simulink model "D2C_boucle_vitesse_modelisation"  (R2018a)
settings: Solver=ode45  StartTime=0.0  StopTime=6  FixedStep=0.003  RelTol=1e-3  EnableMultiTasking=on
settings Model: Creator=Propriétaire  LastModifiedBy=emiliendurif
settings DataIOCC: LimitDataPoints=on  SaveFormat=Array  SignalLoggingSaveFormat=ModelDataLogs
settings OptimizationCC: ExpressionDepthLimit=2147483647  LifeSpan=inf
settings DebuggingCC: UnderspecifiedInitializationDetection=Classic  MergeDetectMultiDrivingBlocksExec=none  SolverPrmCheckMsg=warning  FcnCallInpInsideContextMsg=warning  StateNameClashWarn=warning  SFUnexpectedBacktrackingDiag=warning  SFNoUnconditionalDefaultTransitionDiag=warning  SFExecutionAtInitializationDiag=none
settings HardwareCC: ProdBitPerPointer=32  ProdBitPerSizeT=32  ProdBitPerPtrDiffT=32  ProdLargestAtomicFloat=None  ProdIntDivRoundTo=Undefined  ProdEndianess=Unspecified  ProdWordSize=32  ProdHWDeviceType=32-bit Generic
settings ModelReferenceCC: PropagateSignalLabelsOutOfModel=off
settings CodeAppCC: StateflowObjectComments=on
settings GRTTargetCC: TargetLangStandard=C89/C90 (ANSI)  GeneratePreprocessorConditionals=Disable all  CombineOutputUpdateFcns=off  GRTInterface=on
settings ConfigComp: CovMetricSettings=dw  CovHtmlReporting=on  CovSaveCumulativeToWorkspaceVar=on  CovSaveSingleToWorkspaceVar=on  CovExternalEMLEnable=off

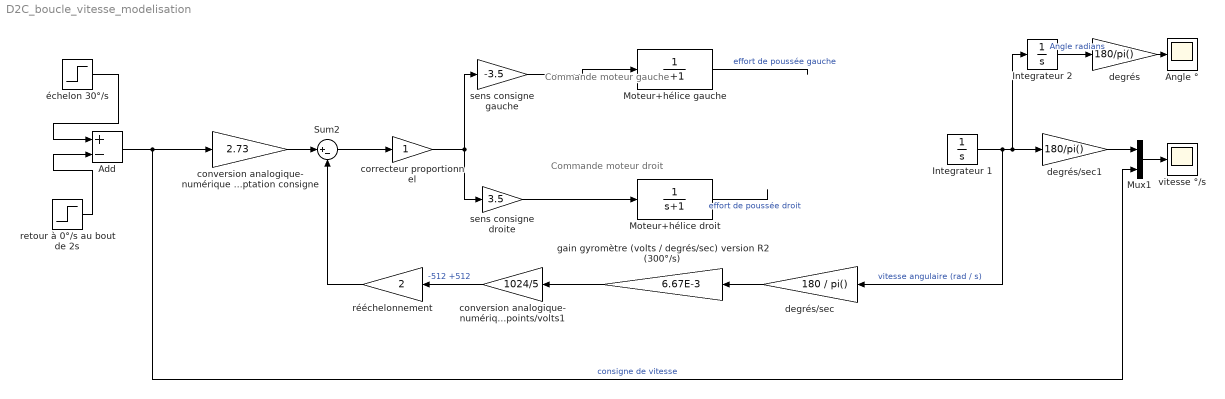
== system D2C_boucle_vitesse_modelisation ==
  note: Commande
      | moteur gauche
  note: Commande
      | moteur droit
  Add : Sum  Inputs=+-
  Angle ° : Scope
  Integrateur 1 : Integrator
  Integrateur 2 : Integrator
  Moteur+hélice droit : TransferFcn  Denominator=[1 1]
  Moteur+hélice gauche : TransferFcn  Denominator=[1 1]
  Mux1 : Mux  Inputs=2
  Sum2 : Sum  Inputs=|+-
  conversion analogique- numérique points/volts 15 bits et adaptation consigne : Gain  Gain=2.73
  conversion analogique- numérique points/volts1 : Gain  Gain=1024/5
  correcteur proportionnel : Gain
  degrés : Gain  Gain=180/pi()
  degrés/sec : Gain  Gain=180 / pi()
  degrés/sec1 : Gain  Gain=180/pi()
  gain gyromètre (volts / degrés/sec) version R2 (300°/s) : Gain  Gain=6.67E-3
  retour à 0°/s au bout de 2s : Step  Time=2  After=30  SampleTime=0
  rééchelonnement : Gain  Gain=2
  sens consigne droite : Gain  Gain=3.5
  sens consigne gauche : Gain  Gain=-3.5
  vitesse °/s : Scope
  échelon 30°/s : Step  Time=0  After=30  SampleTime=0
  wires:
  Moteur+hélice gauche/1 -> ?  "effort de poussée gauche"
  Moteur+hélice droit/1 -> ?  "effort de poussée droit"
  gain gyromètre (volts / degrés/sec) version R2 (300°/s)/1 -> conversion analogique- numérique points/volts1/1
  Integrateur 2/1 -> degrés/1  "Angle radians"
  ? -> Integrateur 1/1  "accélération angulaire"
  Integrateur 1/1 -> Integrateur 2/1, degrés/sec1/1, degrés/sec/1  "vitesse angulaire (rad / s)"
  degrés/sec/1 -> gain gyromètre (volts / degrés/sec) version R2 (300°/s)/1
  degrés/1 -> Angle °/1
  Add/1 -> Mux1/2, conversion analogique- numérique points/volts 15 bits et adaptation consigne/1  "consigne de vitesse"
  degrés/sec1/1 -> Mux1/1
  conversion analogique- numérique points/volts1/1 -> rééchelonnement/1  "-512 +512"
  Mux1/1 -> vitesse °/s/1
  sens consigne droite/1 -> Moteur+hélice droit/1
  sens consigne gauche/1 -> Moteur+hélice gauche/1
  échelon 30°/s/1 -> Add/1
  retour à 0°/s au bout de 2s/1 -> Add/2
  rééchelonnement/1 -> Sum2/2
  conversion analogique- numérique points/volts 15 bits et adaptation consigne/1 -> Sum2/1
  Sum2/1 -> correcteur proportionnel/1
  correcteur proportionnel/1 -> sens consigne gauche/1, sens consigne droite/1
